simulink model "ElectricalFilterWithMultiplePoles"  (R2023b)
settings: Solver=VariableStepAuto  StartTime=0.0  StopTime=20  RelTol=1e-3
values from neighbouring files (symbols this model uses):
  G6_den = [a,b,c,d,e]    [ResonantSystem_ElectricalFilterWithMultiplePoles.m]
  G6_num = [A,B,C,D]    [ResonantSystem_ElectricalFilterWithMultiplePoles.m]
settings Model: Creator=Sofia Katrina Dilag  LastModifiedBy=Sofia Katrina Dilag

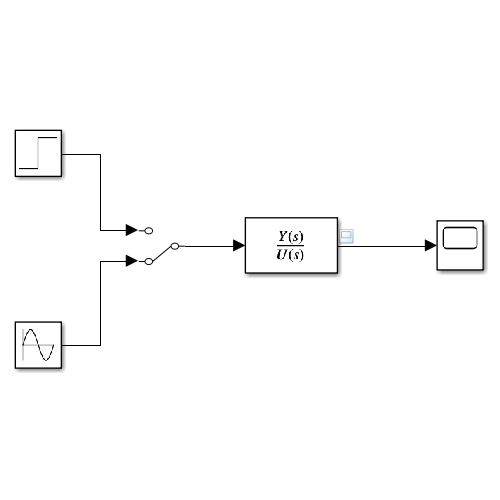
[thumbnail: Simulink's stored preview of the top-level diagram]
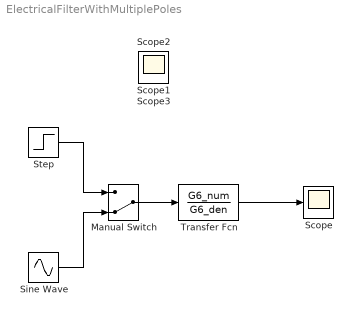
== system ElectricalFilterWithMultiplePoles ==
  Manual Switch : ManualSwitch  CurrentSetting=0
  Scope{,1..3} (4 alike) : Scope
  Sine Wave : Sin  SampleTime=0
  Step : Step  Time=0  Before=0.1  SampleTime=0
  Transfer Fcn : TransferFcn  Numerator=G6_num  Denominator=G6_den  ParameterTunability=Unconstrained
  wires:
  Transfer Fcn/1 -> Scope/1
  Step/1 -> Manual Switch/1
  Sine Wave/1 -> Manual Switch/2
  Manual Switch/1 -> Transfer Fcn/1
